simulink model "Blokdiagram"  (R2019a)
settings: Solver=VariableStepAuto  StartTime=0.0  StopTime=28800  RelTol=1e-3
settings Model: Creator=Anton  LastModifiedBy=Anton
settings SolverCC: AlgebraicLoopSolver=LineSearch

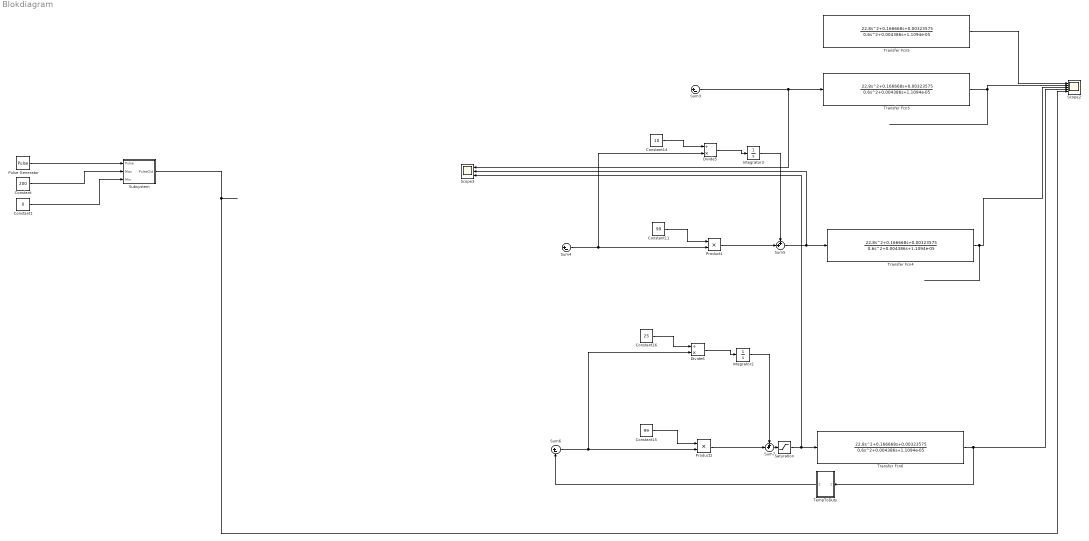
== system Blokdiagram ==
  Constant : Constant  Value=200
  Constant1 : Constant  Value=0
  Constant11 : Constant  Value=99
  Constant14 : Constant  Value=10
  Constant15 : Constant  Value=99
  Constant16 : Constant  Value=25
  Divide5 : Product  Inputs=/*
  Divide6 : Product  Inputs=/*
  Integrator2 : Integrator
  Integrator3 : Integrator
  Product1 : Product
  Product2 : Product
  Pulse Generator : DiscretePulseGenerator  PulseType=Time based  Period=14400  PulseWidth=50  PhaseDelay=7200
  Saturation : Saturate  UpperLimit=1  LowerLimit=0
  Scope2 : Scope  NumInputPorts=5
  Scope3 : Scope  NumInputPorts=3
  Subsystem : Subsystem
  Sum3 : Sum  Inputs=|+-
  Sum4 : Sum  Inputs=|+-
  Sum5 : Sum  Inputs=++|
  Sum6 : Sum  Inputs=|+-
  Sum7 : Sum  Inputs=++|
  TempToDuty : Subsystem
  Transfer Fcn{3..6} (4 alike) : TransferFcn  Numerator=[22.8,0.166668,0.00323575]  Denominator=[0.6,0.004386,1.1094e-05]
  wires:
  Sum3/1 -> Scope3/1, Transfer Fcn3/1
  Transfer Fcn4/1 -> Scope2/3
  Product1/1 -> Sum5/2
  Constant11/1 -> Product1/1
  Transfer Fcn5/1 -> Scope2/1
  Divide5/1 -> Integrator3/1
  Integrator3/1 -> Sum5/1
  Sum4/1 -> Product1/2, Divide5/2
  Constant14/1 -> Divide5/1
  Sum5/1 -> Scope3/2, Transfer Fcn4/1
  Product2/1 -> Sum7/2
  Constant15/1 -> Product2/1
  Transfer Fcn6/1 -> TempToDuty/1(In1), Scope2/4
  Integrator2/1 -> Sum7/1
  Sum6/1 -> Product2/2, Divide6/2
  Sum7/1 -> Saturation/1
  Saturation/1 -> Scope3/3, Transfer Fcn6/1
  Divide6/1 -> Integrator2/1
  Constant16/1 -> Divide6/1
  TempToDuty/1(Out1) -> Sum6/2
  ? -> Sum3/2
  ? -> Transfer Fcn5/1, Sum3/1, Sum6/1, Sum4/1
  Transfer Fcn3/1 -> Scope2/2
  Subsystem/1(PulseOut) -> Scope2/5
  Pulse Generator/1 -> Subsystem/1(Pulse)
  Constant/1 -> Subsystem/2(Max)
  Constant1/1 -> Subsystem/3(Min)
  ? -> Sum4/2

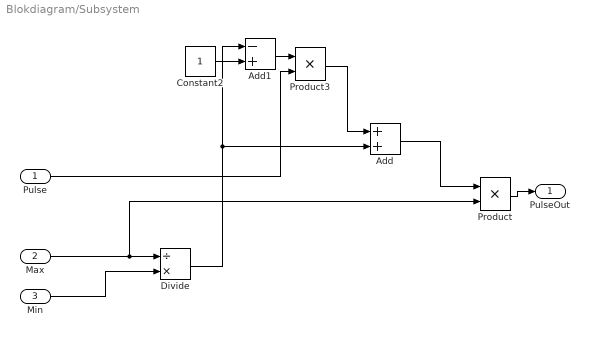
== system Blokdiagram/Subsystem ==
  Pulse : Inport
  Max : Inport  Port=2
  Min : Inport  Port=3
  Add : Sum
  Add1 : Sum  Inputs=-+
  Constant2 : Constant
  Divide : Product  Inputs=/*
  Product : Product
  Product3 : Product
  PulseOut : Outport
  wires:
  Constant2/1 -> Add1/2
  Divide/1 -> Add/2, Add1/1
  Product3/1 -> Add/1
  Max/1 -> Product/2, Divide/1
  Add1/1 -> Product3/1
  Pulse/1 -> Product3/2
  Add/1 -> Product/1
  Min/1 -> Divide/2
  Product/1 -> PulseOut/1

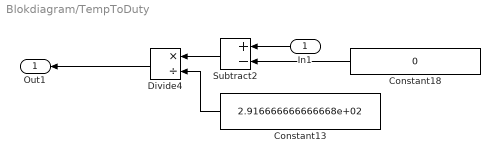
== system Blokdiagram/TempToDuty ==
  In1 : Inport
  Constant13 : Constant  Value=2.916666666666668e+02
  Constant18 : Constant  Value=0
  Divide4 : Product  Inputs=*/
  Subtract2 : Sum  Inputs=+-
  Out1 : Outport
  wires:
  Divide4/1 -> Out1/1
  Subtract2/1 -> Divide4/1
  Constant18/1 -> Subtract2/2
  In1/1 -> Subtract2/1
  Constant13/1 -> Divide4/2
